simulink model "Motor_models"  (R2020b)
settings: Solver=VariableStepAuto  StartTime=0.0  StopTime=10.0  RelTol=1e-3
libraries: autolibmappedmotor x4
settings Model: Creator=True  LastModifiedBy=True

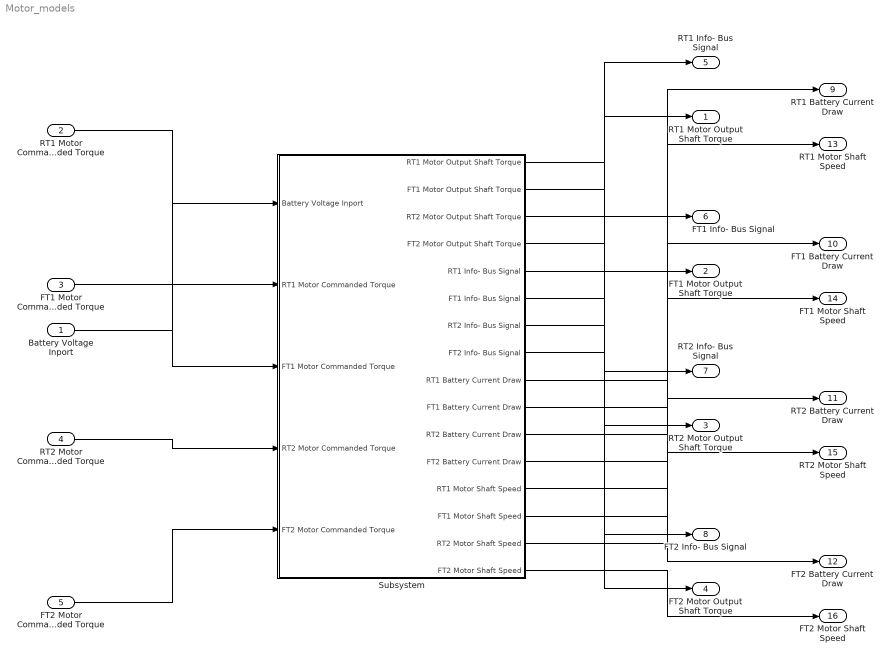
== system Motor_models ==
  Battery Voltage Inport : Inport
  RT1 Motor Commanded Torque : Inport  Port=2
  "FT1 Motor Commanded Torque " : Inport  Port=3
  RT2 Motor Commanded Torque : Inport  Port=4
  FT2 Motor Commanded Torque : Inport  Port=5
  Subsystem : Subsystem
  RT1 Motor Output Shaft Torque : Outport
  FT1 Motor Output Shaft Torque : Outport  Port=2
  RT2 Motor Output Shaft Torque : Outport  Port=3
  FT2 Motor Output Shaft Torque : Outport  Port=4
  RT1 Info- Bus Signal : Outport  Port=5
  FT1 Info- Bus Signal : Outport  Port=6
  RT2 Info- Bus Signal : Outport  Port=7
  FT2 Info- Bus Signal : Outport  Port=8
  RT1 Battery Current Draw : Outport  Port=9
  FT1 Battery Current Draw : Outport  Port=10
  RT2 Battery Current Draw : Outport  Port=11
  FT2 Battery Current Draw : Outport  Port=12
  RT1 Motor Shaft Speed : Outport  Port=13
  FT1 Motor Shaft Speed : Outport  Port=14
  RT2 Motor Shaft Speed : Outport  Port=15
  FT2 Motor Shaft Speed : Outport  Port=16
  wires:
  Battery Voltage Inport/1 -> Subsystem/1(Battery Voltage Inport)
  RT1 Motor Commanded Torque/1 -> Subsystem/2(RT1 Motor Commanded Torque)
  "FT1 Motor Commanded Torque "/1 -> Subsystem/3("FT1 Motor Commanded Torque ")
  RT2 Motor Commanded Torque/1 -> Subsystem/4(RT2 Motor Commanded Torque)
  FT2 Motor Commanded Torque/1 -> Subsystem/5(FT2 Motor Commanded Torque)
  Subsystem/1(RT1 Motor Output Shaft Torque) -> RT1 Motor Output Shaft Torque/1
  Subsystem/2(FT1 Motor Output Shaft Torque) -> FT1 Motor Output Shaft Torque/1
  Subsystem/3(RT2 Motor Output Shaft Torque) -> RT2 Motor Output Shaft Torque/1
  Subsystem/4(FT2 Motor Output Shaft Torque) -> FT2 Motor Output Shaft Torque/1
  Subsystem/5(RT1 Info- Bus Signal) -> RT1 Info- Bus Signal/1
  Subsystem/6(FT1 Info- Bus Signal) -> FT1 Info- Bus Signal/1
  Subsystem/7(RT2 Info- Bus Signal) -> RT2 Info- Bus Signal/1
  Subsystem/8(FT2 Info- Bus Signal) -> FT2 Info- Bus Signal/1
  Subsystem/9(RT1 Battery Current Draw) -> RT1 Battery Current Draw/1
  Subsystem/10(FT1 Battery Current Draw) -> FT1 Battery Current Draw/1
  Subsystem/11(RT2 Battery Current Draw) -> RT2 Battery Current Draw/1
  Subsystem/12(FT2 Battery Current Draw) -> FT2 Battery Current Draw/1
  Subsystem/13(RT1 Motor Shaft Speed) -> RT1 Motor Shaft Speed/1
  Subsystem/14(FT1 Motor Shaft Speed) -> FT1 Motor Shaft Speed/1
  Subsystem/15(RT2 Motor Shaft Speed) -> RT2 Motor Shaft Speed/1
  Subsystem/16(FT2 Motor Shaft Speed) -> FT2 Motor Shaft Speed/1

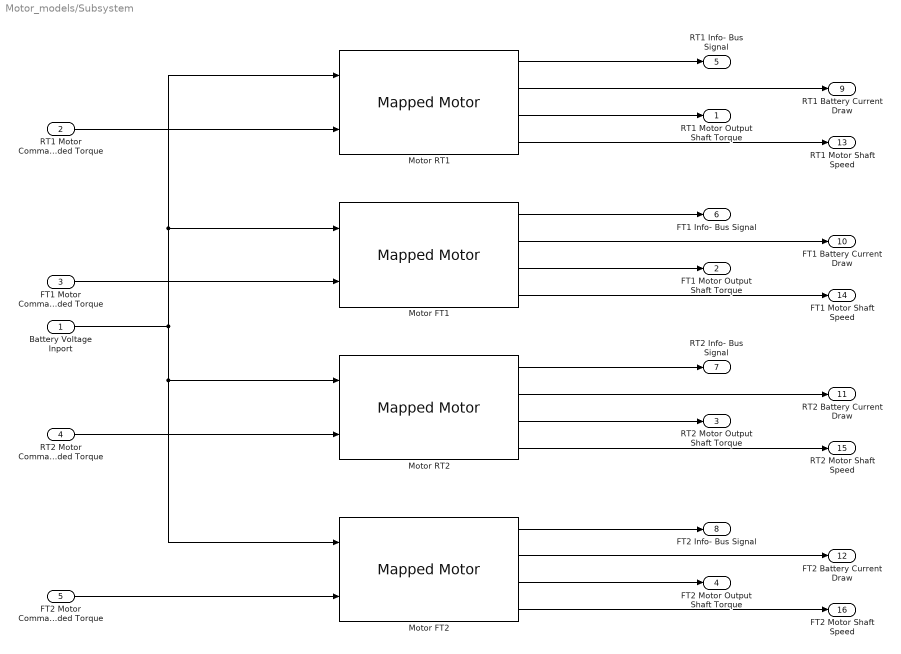
== system Motor_models/Subsystem ==
  Battery Voltage Inport : Inport
  RT1 Motor Commanded Torque : Inport  Port=2
  "FT1 Motor Commanded Torque " : Inport  Port=3
  RT2 Motor Commanded Torque : Inport  Port=4
  FT2 Motor Commanded Torque : Inport  Port=5
  Motor FT1 : autolibmappedmotor/Mapped Motor  port_config=Torque  param_by=Tabulated torque-speed envelope  w_t=[ 0 375 750 800 ]  T_t=[0.09 0.08 0.07 0]  torque_max=.1  power_max=30  Tc=0.02  param_loss=Single efficiency measurement  eff=100  w_eff=375  T_eff=0.08  Piron=0  Pbase=0  w_eff_bp=[-8000 -4000 0 4000 8000]  T_eff_bp=[0 0.03 0.06 0.09]  Temp_eff_bp=[233.15 293.15 373.15]  losses_table=[1.49 1.67 2.21 3.10; 0.42 0.69 1.14 2.03; 0.06 0.24 0.78 1.68; 0.42 0.69 1.14 2.03; 1.49 1.67 2.21 3.10]  losses_table_3d=cat(3,[1.49 1.67 2.21 3.10; 0.42 0.69 1.14 2.03; 0.06 0.24 0.78 1.68; 0.42 0.69 1.14 2.03; 1.49 1.67 2.21 3.10],[1.49 1.67 2.21 3.10; 0.42 0.69 1.14 2.03; 0.06 0.24 0.78 1.68; 0.42 0.69 1.14 2.03; 1.49 1.67 2.21 3.10],[1.49 1.67 2.21 3.10; 0.42 0.69 1.14 2.03; 0.06 0.24 0.78 1.68; 0.42 0.69 1.14 2.03; 1.49 1.67 2.21 3.10])  efficiency_table=[95 95 95 95; 95 95 95 95; 95 95 95 95; 95 95 95 95; 95 95 95 95]  efficiency_table_3d=cat(3,[95 95 95 95; 95 95 95 95; 95 95 95 95; 95 95 95 95; 95 95 95 95],[95 95 95 95; 95 95 95 95; 95 95 95 95; 95 95 95 95; 95 95 95 95],[95 95 95 95; 95 95 95 95; 95 95 95 95; 95 95 95 95; 95 95 95 95])  J=5e-6  b=1e-5  omega_o=0  T_t_extended=[0 0.07 0.08 0.09 0.08 0.07 0]  w_t_extended=[-800 -750 -375 0 375 750 800]  KLossIron=0  KLossCopper=0  x_w_eff_vec=[-8000 -4000 0 4000 8000]  x_T_eff_vec=[-0.09 -0.06 -0.03 0 0.03 0.06 0.09]  x_tmp_eff_vec=[-0.09 -0.06 -0.03 0 0.03 0.06 0.09]  x_losses_mat=[3.1 2.21 1.67 1.49 1.67 2.21 3.1;2.03 1.14 0.69 0.42 0.69 1.14 2.03;1.68 0.78 0.24 0.06 0.24 0.78 1.68;2.03 1.14 0.69 0.42 0.69 1.14 2.03;3.1 2.21 1.67 1.49 1.67 2.21 3.1]  x_losses_mat_3d=[37.8947368421052 25.2631578947368 12.6315789473684 0 12 24 36;18.9473684210526 12.6315789473684 6.3157894736842 0 5.99999999999999 12 18;0 0 0 0 0 0 0;18 12 5.99999999999999 0 6.3157894736842 12.6315789473684 18.9473684210526;36 24 12 0 12.6315789473684 25.2631578947368 37.8947368421052]  CalLossMapData={}  CalLossWithTempMapData={}  aMode=1  RefBlkName='autolibmappedmotor/Mapped Motor'
      settings: SourceProductBaseCode=PW,MT,UV,VE,VP
  Motor FT2 : autolibmappedmotor/Mapped Motor  port_config=Torque  param_by=Tabulated torque-speed envelope  w_t=[ 0 375 750 800 ]  T_t=[0.09 0.08 0.07 0]  torque_max=.1  power_max=30  Tc=0.02  param_loss=Single efficiency measurement  eff=100  w_eff=375  T_eff=0.08  Piron=0  Pbase=0  w_eff_bp=[-8000 -4000 0 4000 8000]  T_eff_bp=[0 0.03 0.06 0.09]  Temp_eff_bp=[233.15 293.15 373.15]  losses_table=[1.49 1.67 2.21 3.10; 0.42 0.69 1.14 2.03; 0.06 0.24 0.78 1.68; 0.42 0.69 1.14 2.03; 1.49 1.67 2.21 3.10]  losses_table_3d=cat(3,[1.49 1.67 2.21 3.10; 0.42 0.69 1.14 2.03; 0.06 0.24 0.78 1.68; 0.42 0.69 1.14 2.03; 1.49 1.67 2.21 3.10],[1.49 1.67 2.21 3.10; 0.42 0.69 1.14 2.03; 0.06 0.24 0.78 1.68; 0.42 0.69 1.14 2.03; 1.49 1.67 2.21 3.10],[1.49 1.67 2.21 3.10; 0.42 0.69 1.14 2.03; 0.06 0.24 0.78 1.68; 0.42 0.69 1.14 2.03; 1.49 1.67 2.21 3.10])  efficiency_table=[95 95 95 95; 95 95 95 95; 95 95 95 95; 95 95 95 95; 95 95 95 95]  efficiency_table_3d=cat(3,[95 95 95 95; 95 95 95 95; 95 95 95 95; 95 95 95 95; 95 95 95 95],[95 95 95 95; 95 95 95 95; 95 95 95 95; 95 95 95 95; 95 95 95 95],[95 95 95 95; 95 95 95 95; 95 95 95 95; 95 95 95 95; 95 95 95 95])  J=5e-6  b=1e-5  omega_o=0  T_t_extended=[0 0.07 0.08 0.09 0.08 0.07 0]  w_t_extended=[-800 -750 -375 0 375 750 800]  KLossIron=0  KLossCopper=0  x_w_eff_vec=[-8000 -4000 0 4000 8000]  x_T_eff_vec=[-0.09 -0.06 -0.03 0 0.03 0.06 0.09]  x_tmp_eff_vec=[-0.09 -0.06 -0.03 0 0.03 0.06 0.09]  x_losses_mat=[3.1 2.21 1.67 1.49 1.67 2.21 3.1;2.03 1.14 0.69 0.42 0.69 1.14 2.03;1.68 0.78 0.24 0.06 0.24 0.78 1.68;2.03 1.14 0.69 0.42 0.69 1.14 2.03;3.1 2.21 1.67 1.49 1.67 2.21 3.1]  x_losses_mat_3d=[37.8947368421052 25.2631578947368 12.6315789473684 0 12 24 36;18.9473684210526 12.6315789473684 6.3157894736842 0 5.99999999999999 12 18;0 0 0 0 0 0 0;18 12 5.99999999999999 0 6.3157894736842 12.6315789473684 18.9473684210526;36 24 12 0 12.6315789473684 25.2631578947368 37.8947368421052]  CalLossMapData={}  CalLossWithTempMapData={}  aMode=1  RefBlkName='autolibmappedmotor/Mapped Motor'
      settings: SourceProductBaseCode=PW,MT,UV,VE,VP
  Motor RT1 : autolibmappedmotor/Mapped Motor  port_config=Torque  param_by=Tabulated torque-speed envelope  w_t=[ 0 375 750 800 ]  T_t=[0.09 0.08 0.07 0]  torque_max=.1  power_max=30  Tc=0.02  param_loss=Single efficiency measurement  eff=100  w_eff=375  T_eff=0.08  Piron=0  Pbase=0  w_eff_bp=[-8000 -4000 0 4000 8000]  T_eff_bp=[0 0.03 0.06 0.09]  Temp_eff_bp=[233.15 293.15 373.15]  losses_table=[1.49 1.67 2.21 3.10; 0.42 0.69 1.14 2.03; 0.06 0.24 0.78 1.68; 0.42 0.69 1.14 2.03; 1.49 1.67 2.21 3.10]  losses_table_3d=cat(3,[1.49 1.67 2.21 3.10; 0.42 0.69 1.14 2.03; 0.06 0.24 0.78 1.68; 0.42 0.69 1.14 2.03; 1.49 1.67 2.21 3.10],[1.49 1.67 2.21 3.10; 0.42 0.69 1.14 2.03; 0.06 0.24 0.78 1.68; 0.42 0.69 1.14 2.03; 1.49 1.67 2.21 3.10],[1.49 1.67 2.21 3.10; 0.42 0.69 1.14 2.03; 0.06 0.24 0.78 1.68; 0.42 0.69 1.14 2.03; 1.49 1.67 2.21 3.10])  efficiency_table=[95 95 95 95; 95 95 95 95; 95 95 95 95; 95 95 95 95; 95 95 95 95]  efficiency_table_3d=cat(3,[95 95 95 95; 95 95 95 95; 95 95 95 95; 95 95 95 95; 95 95 95 95],[95 95 95 95; 95 95 95 95; 95 95 95 95; 95 95 95 95; 95 95 95 95],[95 95 95 95; 95 95 95 95; 95 95 95 95; 95 95 95 95; 95 95 95 95])  J=5e-6  b=1e-5  omega_o=0  T_t_extended=[0 0.07 0.08 0.09 0.08 0.07 0]  w_t_extended=[-800 -750 -375 0 375 750 800]  KLossIron=0  KLossCopper=0  x_w_eff_vec=[-8000 -4000 0 4000 8000]  x_T_eff_vec=[-0.09 -0.06 -0.03 0 0.03 0.06 0.09]  x_tmp_eff_vec=[-0.09 -0.06 -0.03 0 0.03 0.06 0.09]  x_losses_mat=[3.1 2.21 1.67 1.49 1.67 2.21 3.1;2.03 1.14 0.69 0.42 0.69 1.14 2.03;1.68 0.78 0.24 0.06 0.24 0.78 1.68;2.03 1.14 0.69 0.42 0.69 1.14 2.03;3.1 2.21 1.67 1.49 1.67 2.21 3.1]  x_losses_mat_3d=[37.8947368421052 25.2631578947368 12.6315789473684 0 12 24 36;18.9473684210526 12.6315789473684 6.3157894736842 0 5.99999999999999 12 18;0 0 0 0 0 0 0;18 12 5.99999999999999 0 6.3157894736842 12.6315789473684 18.9473684210526;36 24 12 0 12.6315789473684 25.2631578947368 37.8947368421052]  CalLossMapData={}  CalLossWithTempMapData={}  aMode=1  RefBlkName='autolibmappedmotor/Mapped Motor'
      settings: SourceProductBaseCode=PW,MT,UV,VE,VP
  Motor RT2 : autolibmappedmotor/Mapped Motor  port_config=Torque  param_by=Tabulated torque-speed envelope  w_t=[ 0 375 750 800 ]  T_t=[0.09 0.08 0.07 0]  torque_max=.1  power_max=30  Tc=0.02  param_loss=Single efficiency measurement  eff=100  w_eff=375  T_eff=0.08  Piron=0  Pbase=0  w_eff_bp=[-8000 -4000 0 4000 8000]  T_eff_bp=[0 0.03 0.06 0.09]  Temp_eff_bp=[233.15 293.15 373.15]  losses_table=[1.49 1.67 2.21 3.10; 0.42 0.69 1.14 2.03; 0.06 0.24 0.78 1.68; 0.42 0.69 1.14 2.03; 1.49 1.67 2.21 3.10]  losses_table_3d=cat(3,[1.49 1.67 2.21 3.10; 0.42 0.69 1.14 2.03; 0.06 0.24 0.78 1.68; 0.42 0.69 1.14 2.03; 1.49 1.67 2.21 3.10],[1.49 1.67 2.21 3.10; 0.42 0.69 1.14 2.03; 0.06 0.24 0.78 1.68; 0.42 0.69 1.14 2.03; 1.49 1.67 2.21 3.10],[1.49 1.67 2.21 3.10; 0.42 0.69 1.14 2.03; 0.06 0.24 0.78 1.68; 0.42 0.69 1.14 2.03; 1.49 1.67 2.21 3.10])  efficiency_table=[95 95 95 95; 95 95 95 95; 95 95 95 95; 95 95 95 95; 95 95 95 95]  efficiency_table_3d=cat(3,[95 95 95 95; 95 95 95 95; 95 95 95 95; 95 95 95 95; 95 95 95 95],[95 95 95 95; 95 95 95 95; 95 95 95 95; 95 95 95 95; 95 95 95 95],[95 95 95 95; 95 95 95 95; 95 95 95 95; 95 95 95 95; 95 95 95 95])  J=5e-6  b=1e-5  omega_o=0  T_t_extended=[0 0.07 0.08 0.09 0.08 0.07 0]  w_t_extended=[-800 -750 -375 0 375 750 800]  KLossIron=0  KLossCopper=0  x_w_eff_vec=[-8000 -4000 0 4000 8000]  x_T_eff_vec=[-0.09 -0.06 -0.03 0 0.03 0.06 0.09]  x_tmp_eff_vec=[-0.09 -0.06 -0.03 0 0.03 0.06 0.09]  x_losses_mat=[3.1 2.21 1.67 1.49 1.67 2.21 3.1;2.03 1.14 0.69 0.42 0.69 1.14 2.03;1.68 0.78 0.24 0.06 0.24 0.78 1.68;2.03 1.14 0.69 0.42 0.69 1.14 2.03;3.1 2.21 1.67 1.49 1.67 2.21 3.1]  x_losses_mat_3d=[37.8947368421052 25.2631578947368 12.6315789473684 0 12 24 36;18.9473684210526 12.6315789473684 6.3157894736842 0 5.99999999999999 12 18;0 0 0 0 0 0 0;18 12 5.99999999999999 0 6.3157894736842 12.6315789473684 18.9473684210526;36 24 12 0 12.6315789473684 25.2631578947368 37.8947368421052]  CalLossMapData={}  CalLossWithTempMapData={}  aMode=1  RefBlkName='autolibmappedmotor/Mapped Motor'
      settings: SourceProductBaseCode=PW,MT,UV,VE,VP
  RT1 Motor Output Shaft Torque : Outport
  FT1 Motor Output Shaft Torque : Outport  Port=2
  RT2 Motor Output Shaft Torque : Outport  Port=3
  FT2 Motor Output Shaft Torque : Outport  Port=4
  RT1 Info- Bus Signal : Outport  Port=5
  FT1 Info- Bus Signal : Outport  Port=6
  RT2 Info- Bus Signal : Outport  Port=7
  FT2 Info- Bus Signal : Outport  Port=8
  RT1 Battery Current Draw : Outport  Port=9
  FT1 Battery Current Draw : Outport  Port=10
  RT2 Battery Current Draw : Outport  Port=11
  FT2 Battery Current Draw : Outport  Port=12
  RT1 Motor Shaft Speed : Outport  Port=13
  FT1 Motor Shaft Speed : Outport  Port=14
  RT2 Motor Shaft Speed : Outport  Port=15
  FT2 Motor Shaft Speed : Outport  Port=16
  wires:
  Motor FT2/3 -> FT2 Motor Output Shaft Torque/1
  Battery Voltage Inport/1 -> Motor RT2/1, Motor FT2/1, Motor FT1/1, Motor RT1/1
  Motor RT1/1 -> RT1 Info- Bus Signal/1
  RT1 Motor Commanded Torque/1 -> Motor RT1/2
  "FT1 Motor Commanded Torque "/1 -> Motor FT1/2
  Motor RT2/1 -> RT2 Info- Bus Signal/1
  Motor FT1/2 -> FT1 Battery Current Draw/1
  Motor FT1/1 -> FT1 Info- Bus Signal/1
  Motor FT2/1 -> FT2 Info- Bus Signal/1
  Motor FT1/4 -> FT1 Motor Shaft Speed/1
  FT2 Motor Commanded Torque/1 -> Motor FT2/2
  Motor RT2/4 -> RT2 Motor Shaft Speed/1
  Motor RT2/2 -> RT2 Battery Current Draw/1
  Motor FT2/4 -> FT2 Motor Shaft Speed/1
  Motor FT2/2 -> FT2 Battery Current Draw/1
  Motor RT1/3 -> RT1 Motor Output Shaft Torque/1
  RT2 Motor Commanded Torque/1 -> Motor RT2/2
  Motor RT1/4 -> RT1 Motor Shaft Speed/1
  Motor FT1/3 -> FT1 Motor Output Shaft Torque/1
  Motor RT2/3 -> RT2 Motor Output Shaft Torque/1
  Motor RT1/2 -> RT1 Battery Current Draw/1
